simulink model "sih26037_unified_model"  (R2026a)
settings: Solver=ode45  StopTime=10

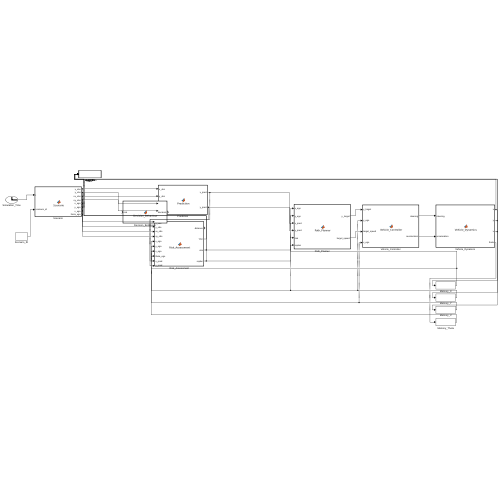
[thumbnail: Simulink's stored preview of the top-level diagram]
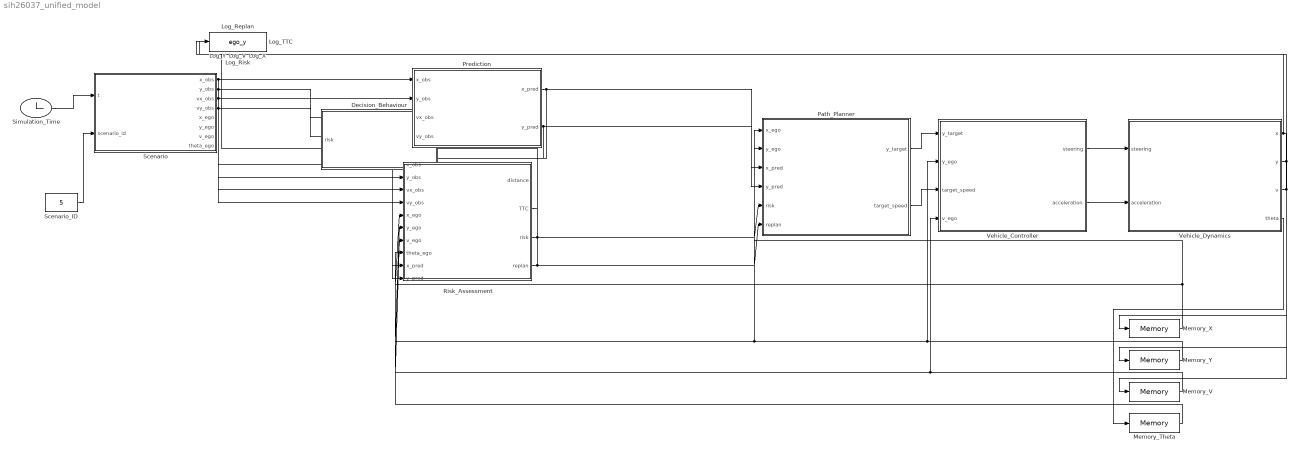
== system sih26037_unified_model ==
  Decision_Behaviour : MATLAB Function  TreatAsAtomicUnit=on
  Log_Replan : ToWorkspace  VariableName=replan_log  SampleTime=-1
  Log_Risk : ToWorkspace  VariableName=risk_log  SampleTime=-1
  Log_TTC : ToWorkspace  VariableName=TTC_log  SampleTime=-1
  Log_V : ToWorkspace  VariableName=ego_v  SampleTime=-1
  Log_X : ToWorkspace  VariableName=ego_x  SampleTime=-1
  Log_Y : ToWorkspace  VariableName=ego_y  SampleTime=-1
  Memory_Theta : Memory
  Memory_V : Memory  InitialCondition=10
  Memory_X : Memory
  Memory_Y : Memory
  Path_Planner : MATLAB Function  TreatAsAtomicUnit=on
  Prediction : MATLAB Function  TreatAsAtomicUnit=on
  Risk_Assessment : MATLAB Function  TreatAsAtomicUnit=on
  Scenario : MATLAB Function  TreatAsAtomicUnit=on
  Scenario_ID : Constant  Value=5
  Simulation_Time : Clock
  Vehicle_Controller : MATLAB Function  TreatAsAtomicUnit=on
  Vehicle_Dynamics : MATLAB Function  TreatAsAtomicUnit=on
  wires:
  Simulation_Time/1 -> Scenario/1(t)
  Scenario/1(x_obs) -> Risk_Assessment/1(x_obs), Prediction/1(x_obs)
  Scenario/2(y_obs) -> Risk_Assessment/2(y_obs), Prediction/2(y_obs)
  Scenario/3(vx_obs) -> Risk_Assessment/3(vx_obs), Prediction/3(vx_obs)
  Scenario/4(vy_obs) -> Risk_Assessment/4(vy_obs), Prediction/4(vy_obs)
  Path_Planner/1(y_target) -> Vehicle_Controller/1(y_target)
  Path_Planner/2(target_speed) -> Vehicle_Controller/3(target_speed)
  Vehicle_Controller/1(steering) -> Vehicle_Dynamics/1(steering)
  Vehicle_Controller/2(acceleration) -> Vehicle_Dynamics/2(acceleration)
  Vehicle_Dynamics/1(x) -> Memory_X/1, Log_X/1
  Vehicle_Dynamics/2(y) -> Memory_Y/1, Log_Y/1
  Vehicle_Dynamics/3(v) -> Memory_V/1, Log_V/1
  Vehicle_Dynamics/4(theta) -> Memory_Theta/1
  Memory_X/1 -> Risk_Assessment/5(x_ego), Path_Planner/1(x_ego)
  Memory_Y/1 -> Risk_Assessment/6(y_ego), Path_Planner/2(y_ego), Vehicle_Controller/2(y_ego)
  Memory_V/1 -> Risk_Assessment/7(v_ego), Vehicle_Controller/4(v_ego)
  Memory_Theta/1 -> Risk_Assessment/8(theta_ego)
  Prediction/1(x_pred) -> Path_Planner/3(x_pred), Risk_Assessment/9(x_pred)
  Prediction/2(y_pred) -> Path_Planner/4(y_pred), Risk_Assessment/10(y_pred)
  Risk_Assessment/3(risk) -> Path_Planner/5(risk), Log_Risk/1
  Risk_Assessment/4(replan) -> Path_Planner/6(replan), Log_Replan/1
  Risk_Assessment/2(TTC) -> Log_TTC/1
  Scenario_ID/1 -> Scenario/2(scenario_id)

== matlab function sih26037_unified_model/Decision_Behaviour ==
  data: risk input; decision output
function decision = Decision_Behaviour(risk)

if risk >= 2
    decision = 2;
elseif risk == 1
    decision = 1;
else
    decision = 0;
end

end

== matlab function sih26037_unified_model/Risk_Assessment ==
  data: distance output; TTC output; risk output; replan output; x_obs input; y_obs input; vx_obs input; vy_obs input; x_ego input; y_ego input; v_ego input; theta_ego input; x_pred input; y_pred input

function [distance,TTC,risk,replan] = Risk_Assessment(x_obs,y_obs,vx_obs,vy_obs,x_ego,y_ego,v_ego,theta_ego,x_pred,y_pred)

predictionTime = 3.0;

% Current relative position
dx = x_obs - x_ego;
dy = y_obs - y_ego;

distance = sqrt(dx*dx + dy*dy);

% Ego velocity
ego_vx = v_ego*cos(theta_ego);
ego_vy = v_ego*sin(theta_ego);

% Current lateral separation
lateralGap = abs(dy);

% Initialize TTC as invalid/no-threat
TTC = 999;

% Longitudinal closing speed
closingSpeedX = ego_vx - vx_obs;

% TTC is meaningful only when obstacle is ahead,
% ego is closing in, and lateral paths overlap

TTC = 999;

if dx > 1.0 && closingSpeedX > 0.001 && lateralGap < 2.5
    TTC = dx / closingSpeedX;
end

% Predict ego position over the same horizon
x_ego_pred = x_ego + ego_vx*predictionTime;
y_ego_pred = y_ego + ego_vy*predictionTime;

% Predicted relative position
predictedDx = x_pred - x_ego_pred;
predictedDy = y_pred - y_ego_pred;

predictedLateralGap = abs(predictedDy);

% Initialize risk
risk = 0;

% Critical risk:
% Obstacle is ahead, lateral paths overlap,
% and predicted/current time gap is short
if (TTC < 2.0 && dx > 0 && lateralGap < 2.5) || ...
        (predictedDx > 0 && predictedDx < 3.0 && predictedLateralGap < 2.5)

    risk = 2;

% Moderate risk
elseif (TTC < 4.0 && dx > 0 && lateralGap < 3.5) || ...
        (predictedDx > 0 && predictedDx < 5.0 && predictedLateralGap < 3.5)

    risk = 1;

end

% Replanning trigger
if risk >= 1
    replan = 1;
else
    replan = 0;
end

end

== matlab function sih26037_unified_model/Scenario ==
  data: t input double size=1; x_obs output double size=1; y_obs output double size=1; vx_obs output double size=1; vy_obs output double size=1; x_ego output double size=1; y_ego output double size=1; v_ego output double size=1; theta_ego output double size=1; scenario_id input double size=1
function [x_obs,y_obs,vx_obs,vy_obs,x_ego,y_ego,v_ego,theta_ego] = Scenario(t,scenario_id)

% Default ego state
x_ego = 0;
y_ego = 0;
theta_ego = 0;

switch scenario_id

    case 1
        % =========================================================
        % UNMARKED VILLAGE ROAD
        % Narrow road with an irregularly moving road user
        % =========================================================
        
        v_ego = 7;

        x_obs = 14 + 0.3*t;
        vx_obs = 0.3;

        if t < 3
            y_obs = 3.0;
            vy_obs = -0.4;

        elseif t < 6
            y_obs = 1.8 - 0.8*(t-3);
            vy_obs = -0.8;

        elseif t < 9
            y_obs = -0.6 + 0.25*(t-6);
            vy_obs = 0.25;

        else
            y_obs = 0.15;
            vy_obs = 0;
        end


    case 2
        % =========================================================
        % URBAN INTERSECTION
        % =========================================================
        
        v_ego = 10;

        x_obs = 12;
        vx_obs = 0;

        if t < 4
            y_obs = 10 - 3*t;
            vy_obs = -3;
        else
            y_obs = -2;
            vy_obs = 0;
        end


    case 3
        % =========================================================
        % HIGHWAY MERGE
        % =========================================================
        
        v_ego = 10;

        x_obs = 18 + 3*t;
        vx_obs = 3;

        if t < 4
            y_obs = 4 - t;
            vy_obs = -1;
        else
            y_obs = 0;
            vy_obs = 0;
        end


    case 4
        % =========================================================
        % DENSE MARKET
        % =========================================================
        
        v_ego = 6;

        x_obs = 10 + 0.5*t;
        vx_obs = 0.5;

        if t < 4
            y_obs = 3 - 0.5*t;
            vy_obs = -0.5;

        elseif t < 7
            y_obs = 1 + 0.3*(t-4);
            vy_obs = 0.3;

        else
            y_obs = 1.9;
            vy_obs = 0;
        end


    case 5
        % =========================================================
        % CATTLE CROSSING
        % =========================================================
        
        v_ego = 8;

        x_obs = 18;
        vx_obs = 0;

        if t < 3
            y_obs = 4.5 - 0.5*t;
            vy_obs = -0.5;

        elseif t < 6
            y_obs = 3 - (t-3);
            vy_obs = -1;

        elseif t < 9
            y_obs = -0.8*(t-6);
            vy_obs = -0.8;

        else
            y_obs = -2.4;
            vy_obs = 0;
        end


    otherwise
        % =========================================================
        % SAFETY DEFAULT
        % =========================================================
        
        v_ego = 10;

        x_obs = 20;
        y_obs = 5;

        vx_obs = 0;
        vy_obs = 0;
end

end

== matlab function sih26037_unified_model/Prediction ==
  data: x_obs input; x_pred output; y_obs input; vx_obs input; vy_obs input; y_pred output
function [x_pred,y_pred] = Prediction(x_obs,y_obs,vx_obs,vy_obs)
 predictionTime = 3.0;
 x_pred = x_obs + vx_obs*predictionTime;
 y_pred = y_obs + vy_obs*predictionTime;
end

== matlab function sih26037_unified_model/Path_Planner ==
  data: x_ego input; y_target output size=1; y_ego input; x_pred input; y_pred input; risk input; replan input; target_speed output size=1
function [y_target,target_speed] = Path_Planner(x_ego,y_ego,x_pred,y_pred,risk,replan)

roadLeft = -4;
roadRight = 4;

% Keep a safety margin from road edges
safeLeft = -2.5;
safeRight = 2.5;

% Default path
y_target = 0;
target_speed = 10;

if replan == 1

    % Conservative candidate paths
    leftPath   = -1.5;
    centerPath = 0;
    rightPath  = 1.5;

    % Calculate distance from predicted obstacle
    clearLeft   = abs(leftPath - y_pred);
    clearCenter = abs(centerPath - y_pred);
    clearRight  = abs(rightPath - y_pred);

    % Prefer a path with greater obstacle separation
    bestClearance = clearLeft;
    y_target = leftPath;

    if clearCenter > bestClearance
        bestClearance = clearCenter;
        y_target = centerPath;
    end

    if clearRight > bestClearance
        bestClearance = clearRight;
        y_target = rightPath;
    end

    % Final safety check
    if y_target < safeLeft
        y_target = safeLeft;
    elseif y_target > safeRight
        y_target = safeRight;
    end

    % Risk-based speed
    if risk >= 2
        target_speed = 3;
    elseif risk == 1
        target_speed = 5;
    else
        target_speed = 7;
    end

end

% Early safety corridor recovery
% Start correcting before reaching the road boundary

if y_ego > 2.0
    y_target = 0;
    target_speed = 4;

elseif y_ego < -2.0
    y_target = 0;
    target_speed = 4;
end

% Emergency boundary protection
if y_ego > 3.0
    y_target = -1.0;
    target_speed = 2;

elseif y_ego < -3.0
    y_target = 1.0;
    target_speed = 2;
end
% EARLY AND STRONG SAFETY CORRECTION

if y_ego > 1.8
    y_target = -1.5;
    target_speed = 2;

elseif y_ego < -1.8
    y_target = 1.5;
    target_speed = 2;
end

% EMERGENCY ROAD-BOUNDARY PROTECTION

if y_ego > 3.0
    y_target = -2.0;
    target_speed = 1;

elseif y_ego < -3.0
    y_target = 2.0;
    target_speed = 1;
end

== matlab function sih26037_unified_model/Vehicle_Controller ==
  data: y_target input; steering output; y_ego input; target_speed input; v_ego input; acceleration output

function [steering,acceleration] = Vehicle_Controller(y_target,y_ego,target_speed,v_ego)

% Controller parameters
Kp = 0.8;
Kd = 0.02;
dt = 0.05;

maxSteering = 0.35;
maxSteeringRate = 0.15;

% Persistent states
persistent previousError previousSteering

if isempty(previousError)
    previousError = 0;
end

if isempty(previousSteering)
    previousSteering = 0;
end

% Lateral error
lateralError = y_target - y_ego;

% Derivative error
derivativeError = (lateralError - previousError) / dt;

% PD steering controller
rawSteering = Kp*lateralError + Kd*derivativeError;

% Boundary safety correction
if y_ego > 3.5 && rawSteering > 0
    rawSteering = -0.2;
elseif y_ego < -3.5 && rawSteering < 0
    rawSteering = 0.2;
end

% Steering saturation
if rawSteering > maxSteering
    rawSteering = maxSteering;
elseif rawSteering < -maxSteering
    rawSteering = -maxSteering;
end

% Strong direct safety correction
if y_ego > 2.0
    rawSteering = -0.35;
elseif y_ego < -2.0
    rawSteering = 0.35;
end

% Steering saturation
if rawSteering > maxSteering
    rawSteering = maxSteering;
elseif rawSteering < -maxSteering
    rawSteering = -maxSteering;
end
% Steering rate limiting
steeringChange = rawSteering - previousSteering;

if steeringChange > maxSteeringRate
    steering = previousSteering + maxSteeringRate;
elseif steeringChange < -maxSteeringRate
    steering = previousSteering - maxSteeringRate;
else
    steering = rawSteering;
end

% Update persistent states
previousError = lateralError;
previousSteering = steering;

% Longitudinal controller
Kv = 0.8;
acceleration = Kv*(target_speed - v_ego);

% Acceleration saturation
if acceleration > 2
    acceleration = 2;
elseif acceleration < -4
    acceleration = -4;
end

end

== matlab function sih26037_unified_model/Vehicle_Dynamics ==
  data: x output; steering input; y output; acceleration input; v output; theta output
function [x,y,v,theta] = Vehicle_Dynamics(steering,acceleration)

% Vehicle parameters
L = 2.7;
dt = 0.05;

% Persistent vehicle state
persistent X Y V THETA

if isempty(X)
    X = 0;
    Y = 0;
    V = 10;
    THETA = 0;
end

% Kinematic vehicle model
X = X + V*cos(THETA)*dt;
Y = Y + V*sin(THETA)*dt;
THETA = THETA + (V/L)*tan(steering)*dt;

% Longitudinal dynamics
V = V + acceleration*dt;

% Prevent negative speed
if V < 0
    V = 0;
end

% Outputs
x = X;
y = Y;
v = V;
theta = THETA;
end
